simulink model "claw_model"  (R2016b)
settings: Solver=FixedStepDiscrete  StartTime=0.0  StopTime=10.0  FixedStep=0.01  RelTol=1e-3
libraries: simulink x2
settings Model: Creator=Borja Martos  LastModifiedBy=Borja Martos

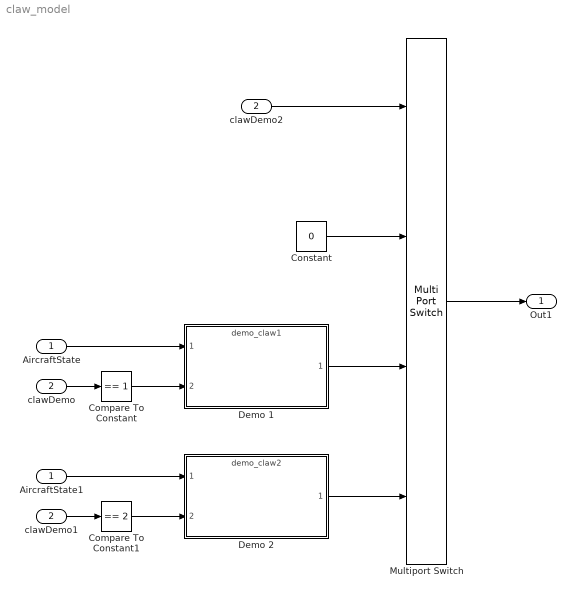
== system claw_model ==
  AircraftState : Inport  OutDataTypeStr=Bus: INPUTS
  clawDemo : Inport  Port=2
  AircraftState1 : InportShadow  OutDataTypeStr=Bus: INPUTS
  Compare To Constant : simulink/Logic and Bit Operations/Compare To Constant  relop===  const=1  OutDataTypeStr=boolean
  Compare To Constant1 : simulink/Logic and Bit Operations/Compare To Constant  relop===  const=2  OutDataTypeStr=boolean
  Constant : Constant  Value=0
  Demo 1 : ModelReference  ModelNameDialog=demo_claw1.slx  SimulationMode=Normal  ModelReferenceVersion=1.6
  Demo 2 : ModelReference  ModelNameDialog=demo_claw2.slx  SimulationMode=Normal  ModelReferenceVersion=1.7
  Multiport Switch : MultiPortSwitch  DataPortOrder=Zero-based contiguous  DiagnosticForDefault=None
  clawDemo1 : InportShadow  Port=2
  clawDemo2 : InportShadow  Port=2
  Out1 : Outport
  wires:
  AircraftState/1 -> Demo 1/1
  clawDemo/1 -> Compare To Constant/1
  Compare To Constant/1 -> Demo 1/2
  AircraftState1/1 -> Demo 2/1
  clawDemo1/1 -> Compare To Constant1/1
  Compare To Constant1/1 -> Demo 2/2
  Demo 2/1 -> Multiport Switch/4
  clawDemo2/1 -> Multiport Switch/1
  Multiport Switch/1 -> Out1/1
  Demo 1/1 -> Multiport Switch/3
  Constant/1 -> Multiport Switch/2
